simulink model "physicsSPD"  (R2015a)
settings: Solver=ode45  StartTime=0.0  StopTime=10.0  RelTol=1e-3
values from neighbouring files (symbols this model uses):
  Kd = .5*rho*Cd*A    (= 600)    [depth_ctl_design.m]
undefined symbols (not defined in the file or in its folder): mass
libraries: simulink x2
settings Model: Creator=Cassandra  LastModifiedBy=Cassandra

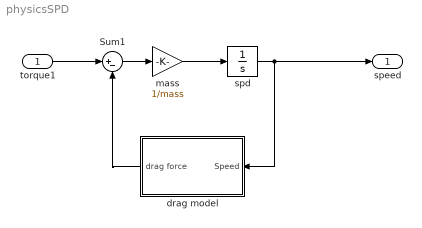
== system physicsSPD ==
  torque1 : Inport
  Sum1 : Sum  Inputs=|+-
  drag model : Subsystem
  mass : Gain  Gain=1/mass
  spd : Integrator
  speed : Outport
  wires:
  mass/1 -> spd/1
  spd/1 -> speed/1, drag model/1(Speed)
  Sum1/1 -> mass/1
  drag model/1(drag force) -> Sum1/2
  torque1/1 -> Sum1/1

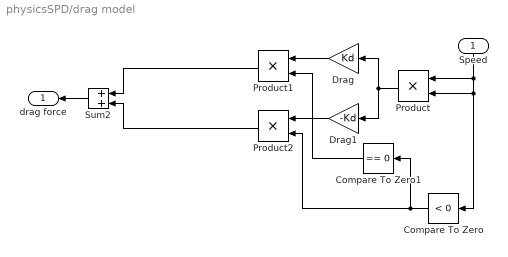
== system physicsSPD/drag model ==
  Speed : Inport
  Compare To Zero : simulink/Logic and Bit Operations/Compare To Zero  relop=<  OutDataTypeStr=boolean
  Compare To Zero1 : simulink/Logic and Bit Operations/Compare To Zero  relop===  OutDataTypeStr=boolean
  Drag : Gain  Gain=Kd
  Drag1 : Gain  Gain=-Kd
  Product : Product
  Product1 : Product
  Product2 : Product
  Sum2 : Sum  Inputs=+|+
  drag force : Outport
  wires:
  Speed/1 -> Product/1, Compare To Zero/1, Product/2
  Drag1/1 -> Product2/1
  Compare To Zero1/1 -> Product1/2
  Product1/1 -> Sum2/1
  Drag/1 -> Product1/1
  Sum2/1 -> drag force/1
  Product/1 -> Drag1/1, Drag/1
  Product2/1 -> Sum2/2
  Compare To Zero/1 -> Product2/2, Compare To Zero1/1
